simulink library "lib_subframe_20a"  (R2020a)
settings: Solver=VariableStepAuto  StartTime=0.0  StopTime=10.0  RelTol=1e-3
libraries: xpcutilitieslib x1
settings Model: Creator=jiw19031  LastModifiedBy=mrajase
settings DebuggingCC: SFMachineParentedDataDiag=error

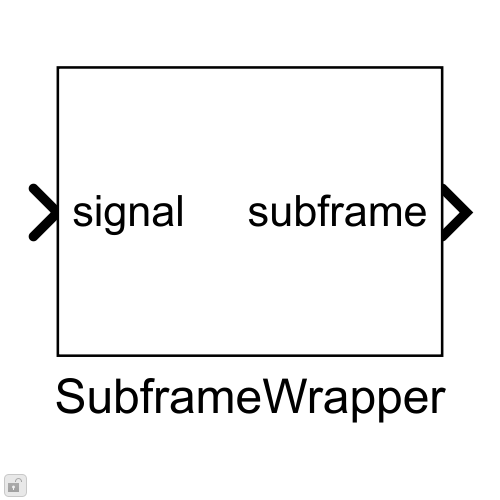
[thumbnail: Simulink's stored preview of the top-level diagram]
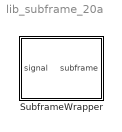
== system lib_subframe_20a ==
  SubframeWrapper : Subsystem  mask{data_id=1}

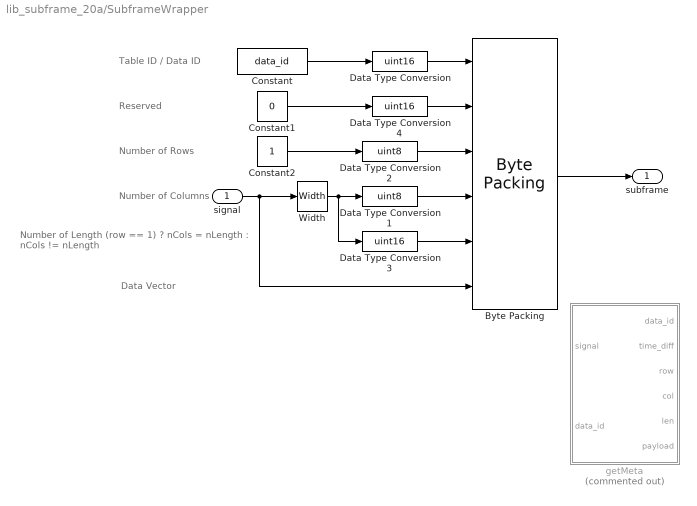
== system lib_subframe_20a/SubframeWrapper ==
  note: Table ID / Data ID
  note: Reserved
  note: Number of Rows
  note: Number of Columns
  note: Number of Length
      | (row == 1) ? nCols = nLength : nCols != nLength
  note: Data Vector
  signal : Inport
  "Byte Packing " : xpcutilitieslib/Byte Packing   MaskPackedDataType=uint8  MaskUnpackedDataTypes={'uint16','uint16','uint8','uint8','uint16','double'}  MaskAlignment=1
  Constant : Constant  Value=data_id
  Constant1 : Constant  Value=0
  Constant2 : Constant
  Data Type Conversion : DataTypeConversion  OutDataTypeStr=uint16
  Data Type Conversion1 : DataTypeConversion  OutDataTypeStr=uint8
  Data Type Conversion2 : DataTypeConversion  OutDataTypeStr=uint8
  Data Type Conversion3 : DataTypeConversion  OutDataTypeStr=uint16
  Data Type Conversion4 : DataTypeConversion  OutDataTypeStr=uint16
  Width : Width
  getMeta : MATLAB Function  Commented=on  TreatAsAtomicUnit=on
  subframe : Outport
  wires:
  Constant/1 -> Data Type Conversion/1
  "Byte Packing "/1 -> subframe/1
  Constant2/1 -> Data Type Conversion2/1
  Constant1/1 -> Data Type Conversion4/1
  Width/1 -> Data Type Conversion3/1, Data Type Conversion1/1
  Data Type Conversion2/1 -> "Byte Packing "/3
  Data Type Conversion1/1 -> "Byte Packing "/4
  Data Type Conversion4/1 -> "Byte Packing "/2
  Data Type Conversion3/1 -> "Byte Packing "/5
  Data Type Conversion/1 -> "Byte Packing "/1
  signal/1 -> "Byte Packing "/6, Width/1

== matlab function lib_subframe_20a/SubframeWrapper/getMeta ==
  data: data_id output; time_diff output; row output; col output; len output; signal input; payload output; data_id input
function [ data_id,time_diff,row,col,len, payload]=get_meta(signal, data_id)
[row, col]=size(signal);
len = row*col;
time_diff = 0;
payload = signal;
